simulink model "test_sys"  (R2016b)
settings: Solver=VariableStepAuto  StartTime=0.0  StopTime=100  RelTol=1e-3
libraries: simulink x2
settings Model: Creator=Sky  LastModifiedBy=Sky

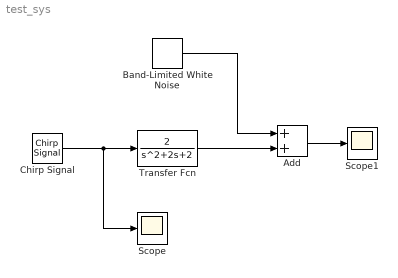
== system test_sys ==
  Add : Sum
  Band-Limited White Noise : simulink/Sources/Band-Limited White Noise  Cov=[0.000001]  Ts=0.1  seed=[23341]
  Chirp Signal : simulink/Sources/Chirp Signal  f1=0.001  T=100  f2=3
  Scope : Scope
  Scope1 : Scope
  Transfer Fcn : TransferFcn  Numerator=[2]  Denominator=[1 2 2]
  wires:
  Chirp Signal/1 -> Scope/1, Transfer Fcn/1
  Transfer Fcn/1 -> Add/2
  Band-Limited White Noise/1 -> Add/1
  Add/1 -> Scope1/1
